simulink subsystem "Batter_Pack_Sim"  (R2022b)
settings: Solver=VariableStepAuto  StartTime=0.0  StopTime=10.0  RelTol=1e-3
undefined symbols (not defined in the file or in its folder): BATT, C, Ion, Lithium, R
libraries: spsIdealSwitchLib x9, spsParallelRLCBranchLib x6, spsBatteryLib x3
settings Model: Creator=MAAM  LastModifiedBy=MAAM

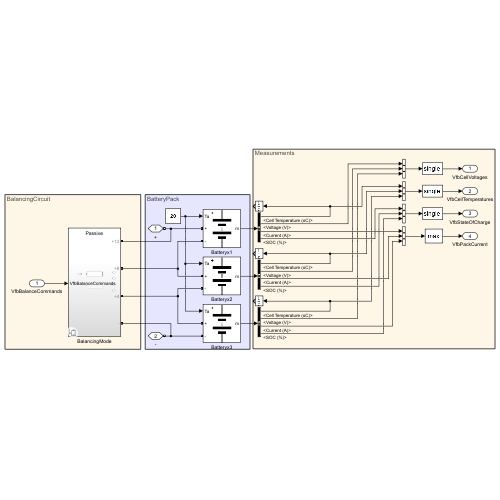
[thumbnail: Simulink's stored preview of the top-level diagram]
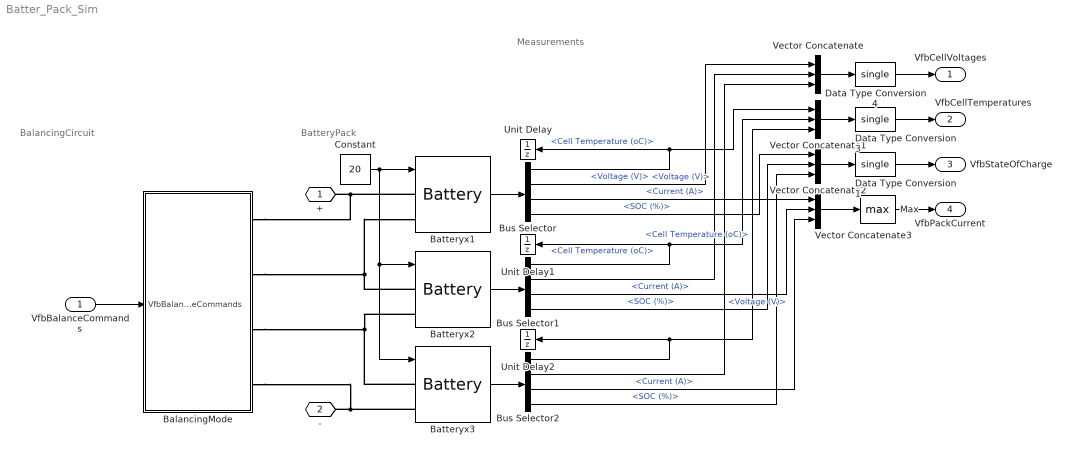
== system Batter_Pack_Sim ==
  note: BalancingCircuit
  note: Measurements
  note: BatteryPack
  VfbBalanceCommands : Inport
  BalancingMode : Subsystem  Variant=on
  Batteryx1 : spsBatteryLib/Battery  BatType=Lithium-Ion  ShowTempParam=on  ThermalPreset=no  ShowAgeParam=off  NomV=double(BATT.Voltage.NominalVolt)  NomQ=double(BATT.Capacity.Type)  SOC=75  Batt_Tr=30  PresetModel=off  MaxQ=double(BATT.Capacity.Max)  MinV=2.55  FullV=double(BATT.Voltage.Full_Dchrg)  Dis_rate=1.3043  R=double(BATT.Res.R0)  Normal_OP=double(BATT.Capacity.Rate)  expZone="[4     0.34]"  current=[6.5 13 32.5]  Units=Time  Tci=20  NomT=20  T2=-30  MaxQ2=double(BATT.Capacity.Rate)  FullV2=double(BATT.Voltage.Init_Dchrg)  Normal_OP2=2.75  expZone2=[3.25 0.5]  Rca=0.06  ti=1000  Dp=0  Neq0=0  Tsim=1e6  Ta1=25  Qeol=5.4*0.9  Reol=0.013333*1.2  Char_age=[2.3478, 3]  Dis_age=[2.3478, 10]  N1=1500  N2=10500  N3=1000  N4=1400  Ta2=45  N5=950
  Batteryx2 : spsBatteryLib/Battery  BatType=Lithium-Ion  ShowTempParam=on  ThermalPreset=no  ShowAgeParam=off  NomV=double(BATT.Voltage.NominalVolt)  NomQ=double(BATT.Capacity.Type)  SOC=85  Batt_Tr=30  PresetModel=off  MaxQ=double(BATT.Capacity.Max)  MinV=2.55  FullV=double(BATT.Voltage.Full_Dchrg)  Dis_rate=1.3043  R=double(BATT.Res.R0)  Normal_OP=double(BATT.Capacity.Rate)  expZone="[4     0.34]"  current=[6.5 13 32.5]  Units=Time  Tci=20  NomT=20  T2=-30  MaxQ2=double(BATT.Capacity.Rate)  FullV2=double(BATT.Voltage.Init_Dchrg)  Normal_OP2=2.75  expZone2=[3.25 0.5]  Rca=0.06  ti=1000  Dp=0  Neq0=0  Tsim=1e6  Ta1=25  Qeol=5.4*0.9  Reol=0.013333*1.2  Char_age=[2.3478, 3]  Dis_age=[2.3478, 10]  N1=1500  N2=10500  N3=1000  N4=1400  Ta2=45  N5=950
  Batteryx3 : spsBatteryLib/Battery  BatType=Lithium-Ion  ShowTempParam=on  ThermalPreset=no  ShowAgeParam=off  NomV=double(BATT.Voltage.NominalVolt)  NomQ=double(BATT.Capacity.Type)  SOC=65  Batt_Tr=30  PresetModel=off  MaxQ=double(BATT.Capacity.Max)  MinV=2.55  FullV=double(BATT.Voltage.Full_Dchrg)  Dis_rate=1.3043  R=double(BATT.Res.R0)  Normal_OP=double(BATT.Capacity.Rate)  expZone="[4     0.34]"  current=[6.5 13 32.5]  Units=Time  Tci=20  NomT=20  T2=-30  MaxQ2=double(BATT.Capacity.Rate)  FullV2=double(BATT.Voltage.Init_Dchrg)  Normal_OP2=2.75  expZone2=[3.25 0.5]  Rca=0.06  ti=1000  Dp=0  Neq0=0  Tsim=1e6  Ta1=25  Qeol=5.4*0.9  Reol=0.013333*1.2  Char_age=[2.3478, 3]  Dis_age=[2.3478, 10]  N1=1500  N2=10500  N3=1000  N4=1400  Ta2=45  N5=950
  Bus Selector : BusSelector  OutputSignals=Cell Temperature (oC),Voltage (V),Current (A),SOC (%)
  Bus Selector1 : BusSelector  OutputSignals=Cell Temperature (oC),Voltage (V),Current (A),SOC (%)
  Bus Selector2 : BusSelector  OutputSignals=Cell Temperature (oC),Voltage (V),Current (A),SOC (%)
  Constant : Constant  Value=20
  Data Type Conversion1 : DataTypeConversion  OutDataTypeStr=single  SaturateOnIntegerOverflow=off  RndMeth=Floor
  Data Type Conversion3 : DataTypeConversion  OutDataTypeStr=single  SaturateOnIntegerOverflow=off  RndMeth=Floor
  Data Type Conversion4 : DataTypeConversion  OutDataTypeStr=single  SaturateOnIntegerOverflow=off  RndMeth=Floor
  Max : MinMax  Function=max  OutDataTypeStr=single
  Unit Delay : UnitDelay  InitialCondition=20  SampleTime=-1  HasFrameUpgradeWarning=on
  Unit Delay1 : UnitDelay  InitialCondition=20  SampleTime=-1  HasFrameUpgradeWarning=on
  Unit Delay2 : UnitDelay  InitialCondition=20  SampleTime=-1  HasFrameUpgradeWarning=on
  Vector Concatenate{,1..3} (4 alike) : Concatenate  NumInputs=3
  + : PMIOPort  Side=Left
  - : PMIOPort  Port=2  Side=Left
  VfbCellVoltages : Outport
  VfbCellTemperatures : Outport  Port=2
  VfbStateOfCharge : Outport  Port=3
  VfbPackCurrent : Outport  Port=4
  wires:
  Constant/1 -> Batteryx2/1, Batteryx3/1, Batteryx1/1
  Data Type Conversion4/1 -> VfbCellVoltages/1
  Data Type Conversion3/1 -> VfbCellTemperatures/1
  Data Type Conversion1/1 -> VfbStateOfCharge/1
  Max/1 -> VfbPackCurrent/1
  Bus Selector1/3 -> Vector Concatenate3/2  "<Current (A)>"
  Bus Selector2/1 -> Vector Concatenate1/3, Unit Delay2/1  "<Cell Temperature (oC)>"
  Bus Selector1/2 -> Vector Concatenate/2  "<Voltage (V)>"
  Vector Concatenate3/1 -> Max/1
  Batteryx1/1 -> Bus Selector/1
  Bus Selector1/4 -> Vector Concatenate2/2  "<SOC (%)>"
  Bus Selector1/1 -> Vector Concatenate1/2, Unit Delay1/1  "<Cell Temperature (oC)>"
  Batteryx3/1 -> Bus Selector2/1
  Bus Selector/4 -> Vector Concatenate2/1  "<SOC (%)>"
  Vector Concatenate2/1 -> Data Type Conversion1/1
  Vector Concatenate/1 -> Data Type Conversion4/1
  Bus Selector2/4 -> Vector Concatenate2/3  "<SOC (%)>"
  Bus Selector/2 -> Vector Concatenate/1  "<Voltage (V)>"
  Bus Selector/3 -> Vector Concatenate3/1  "<Current (A)>"
  Vector Concatenate1/1 -> Data Type Conversion3/1
  Bus Selector2/3 -> Vector Concatenate3/3  "<Current (A)>"
  Batteryx2/1 -> Bus Selector1/1
  Bus Selector2/2 -> Vector Concatenate/3  "<Voltage (V)>"
  Bus Selector/1 -> Vector Concatenate1/1, Unit Delay/1  "<Cell Temperature (oC)>"
  VfbBalanceCommands/1 -> BalancingMode/1(VfbBalanceCommands)
  connections:
  +/RConn1 -- Batteryx1/LConn1 -- BalancingMode/RConn1
  Batteryx3/LConn1 -- BalancingMode/RConn3 -- Batteryx2/LConn2
  Batteryx2/LConn1 -- BalancingMode/RConn2 -- Batteryx1/LConn2
  Batteryx3/LConn2 -- BalancingMode/RConn4 -- -/RConn1

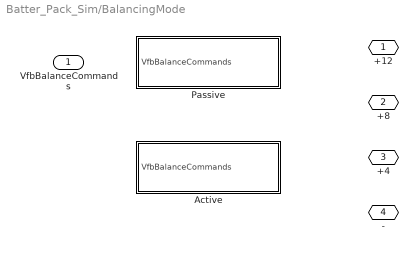
== system Batter_Pack_Sim/BalancingMode ==
  VfbBalanceCommands : Inport
  Active : Subsystem  VariantControl=BATT.Balancing.Mode == BMS_BalMode_Enum.BMS_Active
  Passive : Subsystem  VariantControl=BATT.Balancing.Mode == BMS_BalMode_Enum.BMS_Passive
  +12 : PMIOPort  Side=Right
  +8 : PMIOPort  Port=2  Side=Right
  +4 : PMIOPort  Port=3  Side=Right
  - : PMIOPort  Port=4  Side=Right

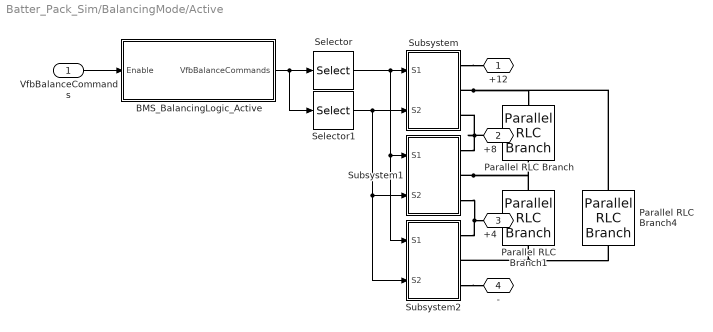
== system Batter_Pack_Sim/BalancingMode/Active ==
  VfbBalanceCommands : Inport
  BMS_BalancingLogic_Active : Stateflow chart  TreatAsAtomicUnit=on
  Parallel RLC Branch : spsParallelRLCBranchLib/Parallel RLC Branch  LConnTagsString=a  RConnTagsString=__new0  BranchType=C  Resistance=1  Inductance=1e-3  SetiL0=off  InitialCurrent=0  Capacitance=C  Setx0=off  InitialVoltage=0  Measurements=None
  Parallel RLC Branch1 : spsParallelRLCBranchLib/Parallel RLC Branch  LConnTagsString=a  RConnTagsString=__new0  BranchType=C  Resistance=1  Inductance=1e-3  SetiL0=off  InitialCurrent=0  Capacitance=C  Setx0=off  InitialVoltage=0  Measurements=None
  Parallel RLC Branch4 : spsParallelRLCBranchLib/Parallel RLC Branch  LConnTagsString=a  RConnTagsString=__new0  BranchType=C  Resistance=1  Inductance=1e-3  SetiL0=off  InitialCurrent=0  Capacitance=C  Setx0=off  InitialVoltage=0  Measurements=None
  Selector : Selector  InputPortWidth=3  IndexOptions=Index vector (dialog)  Indices=1  OutputSizes=1
  Selector1 : Selector  InputPortWidth=3  IndexOptions=Index vector (dialog)  Indices=2  OutputSizes=1
  Subsystem : Subsystem
  Subsystem1 : Subsystem
  Subsystem2 : Subsystem
  +12 : PMIOPort  Side=Right
  +8 : PMIOPort  Port=2  Side=Right
  +4 : PMIOPort  Port=3  Side=Right
  - : PMIOPort  Port=4  Side=Right
  wires:
  Selector1/1 -> Subsystem/2(S2), Subsystem1/2(S2), Subsystem2/2(S2)
  BMS_BalancingLogic_Active/1(VfbBalanceCommands) -> Selector1/1, Selector/1
  Selector/1 -> Subsystem2/1(S1), Subsystem1/1(S1), Subsystem/1(S1)
  VfbBalanceCommands/1 -> BMS_BalancingLogic_Active/1(Enable)
  connections:
  Subsystem1/RConn2 -- Parallel RLC Branch1/LConn1 -- Parallel RLC Branch/RConn1
  Subsystem1/RConn3 -- Subsystem2/RConn1 -- +4/RConn1
  Subsystem/RConn2 -- Parallel RLC Branch4/LConn1 -- Parallel RLC Branch/LConn1
  +8/RConn1 -- Subsystem/RConn3 -- Subsystem1/RConn1
  Parallel RLC Branch1/RConn1 -- Parallel RLC Branch4/RConn1 -- Subsystem2/RConn2
  Subsystem2/RConn3 -- -/RConn1
  Subsystem/RConn1 -- +12/RConn1

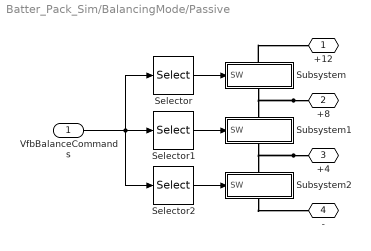
== system Batter_Pack_Sim/BalancingMode/Passive ==
  VfbBalanceCommands : Inport
  Selector : Selector  InputPortWidth=3  IndexOptions=Index vector (dialog)  Indices=1  OutputSizes=1
  Selector1 : Selector  InputPortWidth=3  IndexOptions=Index vector (dialog)  Indices=2  OutputSizes=1
  Selector2 : Selector  InputPortWidth=3  IndexOptions=Index vector (dialog)  Indices=3  OutputSizes=1
  Subsystem : Subsystem
      settings: PortSchema="{\"entries\":[{\"content\":{\"sides\":[{\"content\":{\"connectorIds\":[\"LConn1\"]},\"type\":\"ConnectorPlacement.EquallySpacedRectSide\",\"uuid\":\"eb8fffcd-a71c-4890-8fe1-844de9bb7049\"},{\"content\":{\"connectorIds\":[\"RConn1\"],\"side\":\"RIGHT\"},\"type\":\"ConnectorPlacement.EquallySpacedRectSide\",\"uuid\":\"5d4b0459-fb12-4785-8c10-98c9b0dba58c\"},{\"content\":{\"connectorIds\":[],\"side\":\"TOP\"},\"type\":\"ConnectorPlacement.EquallySpacedRectSide\",\"uuid\":\"54a7a206-2e51-43a0-a96b-a7248b1ad494\"},{\"content\":{\"connectorIds\":[\"In1\"],\"side\":\"BOTTOM\"},\"type\":\"ConnectorPlacement.EquallySpacedRectSide\",\"uuid\":\"fc2549f3-9c78-4be1-a150-7df7a886db86\"}]},\"type\":\"ConnectorPlacement.EquallySpacedConnector\",\"uuid\":\"ba80d02d-3106-485f-afc0-f5d68efbd5a7\"}],\"packageUris\":[\"http://schema.mathworks.com/mf0/Connector/R2020b\"],\"version\":\"1.0\"}"
  Subsystem1 : Subsystem
      settings: PortSchema="{\"entries\":[{\"content\":{\"sides\":[{\"content\":{\"connectorIds\":[\"LConn1\"]},\"type\":\"ConnectorPlacement.EquallySpacedRectSide\",\"uuid\":\"eb8fffcd-a71c-4890-8fe1-844de9bb7049\"},{\"content\":{\"connectorIds\":[\"RConn1\"],\"side\":\"RIGHT\"},\"type\":\"ConnectorPlacement.EquallySpacedRectSide\",\"uuid\":\"5d4b0459-fb12-4785-8c10-98c9b0dba58c\"},{\"content\":{\"connectorIds\":[],\"side\":\"TOP\"},\"type\":\"ConnectorPlacement.EquallySpacedRectSide\",\"uuid\":\"54a7a206-2e51-43a0-a96b-a7248b1ad494\"},{\"content\":{\"connectorIds\":[\"In1\"],\"side\":\"BOTTOM\"},\"type\":\"ConnectorPlacement.EquallySpacedRectSide\",\"uuid\":\"e038b7f9-73dc-4924-8410-20e90d9da844\"}]},\"type\":\"ConnectorPlacement.EquallySpacedConnector\",\"uuid\":\"ba80d02d-3106-485f-afc0-f5d68efbd5a7\"}],\"packageUris\":[\"http://schema.mathworks.com/mf0/Connector/R2020b\"],\"version\":\"1.0\"}"
  Subsystem2 : Subsystem
      settings: PortSchema="{\"entries\":[{\"content\":{\"sides\":[{\"content\":{\"connectorIds\":[\"LConn1\"]},\"type\":\"ConnectorPlacement.EquallySpacedRectSide\",\"uuid\":\"eb8fffcd-a71c-4890-8fe1-844de9bb7049\"},{\"content\":{\"connectorIds\":[\"RConn1\"],\"side\":\"RIGHT\"},\"type\":\"ConnectorPlacement.EquallySpacedRectSide\",\"uuid\":\"5d4b0459-fb12-4785-8c10-98c9b0dba58c\"},{\"content\":{\"connectorIds\":[],\"side\":\"TOP\"},\"type\":\"ConnectorPlacement.EquallySpacedRectSide\",\"uuid\":\"54a7a206-2e51-43a0-a96b-a7248b1ad494\"},{\"content\":{\"connectorIds\":[\"In1\"],\"side\":\"BOTTOM\"},\"type\":\"ConnectorPlacement.EquallySpacedRectSide\",\"uuid\":\"f8f2bbaf-62e5-4d8f-96ff-782bcab3079c\"}]},\"type\":\"ConnectorPlacement.EquallySpacedConnector\",\"uuid\":\"ba80d02d-3106-485f-afc0-f5d68efbd5a7\"}],\"packageUris\":[\"http://schema.mathworks.com/mf0/Connector/R2020b\"],\"version\":\"1.0\"}"
  +12 : PMIOPort  Side=Right
  +8 : PMIOPort  Port=2  Side=Right
  +4 : PMIOPort  Port=3  Side=Right
  - : PMIOPort  Port=4  Side=Right
  wires:
  VfbBalanceCommands/1 -> Selector2/1, Selector/1, Selector1/1
  Selector/1 -> Subsystem/1(SW)
  Selector1/1 -> Subsystem1/1(SW)
  Selector2/1 -> Subsystem2/1(SW)
  connections:
  +4/RConn1 -- Subsystem2/LConn1 -- Subsystem1/RConn1
  +8/RConn1 -- Subsystem1/LConn1 -- Subsystem/RConn1
  Subsystem/LConn1 -- +12/RConn1
  Subsystem2/RConn1 -- -/RConn1

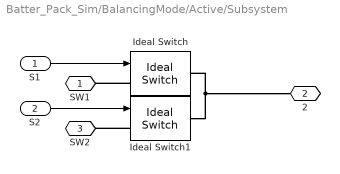
== system Batter_Pack_Sim/BalancingMode/Active/Subsystem ==
  S1 : Inport
  S2 : Inport  Port=2
  Ideal Switch : spsIdealSwitchLib/Ideal Switch  Ron=0.0001  Lon=0  IC=0  Rs=1e7  Cs=inf  Measurements=off
  Ideal Switch1 : spsIdealSwitchLib/Ideal Switch  Ron=0.0001  Lon=0  IC=0  Rs=1e7  Cs=inf  Measurements=off
  SW1 : PMIOPort  Side=Right
  2 : PMIOPort  Port=2  Side=Right
  SW2 : PMIOPort  Port=3  Side=Right
  wires:
  S1/1 -> Ideal Switch/1
  S2/1 -> Ideal Switch1/1
  connections:
  Ideal Switch1/RConn1 -- 2/RConn1 -- Ideal Switch/RConn1
  Ideal Switch/LConn1 -- SW1/RConn1
  Ideal Switch1/LConn1 -- SW2/RConn1

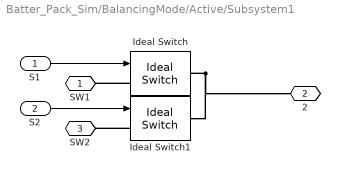
== system Batter_Pack_Sim/BalancingMode/Active/Subsystem1 ==
  S1 : Inport
  S2 : Inport  Port=2
  Ideal Switch : spsIdealSwitchLib/Ideal Switch  Ron=0.0001  Lon=0  IC=0  Rs=1e7  Cs=inf  Measurements=off
  Ideal Switch1 : spsIdealSwitchLib/Ideal Switch  Ron=0.0001  Lon=0  IC=0  Rs=1e7  Cs=inf  Measurements=off
  SW1 : PMIOPort  Side=Right
  2 : PMIOPort  Port=2  Side=Right
  SW2 : PMIOPort  Port=3  Side=Right
  wires:
  S2/1 -> Ideal Switch1/1
  S1/1 -> Ideal Switch/1
  connections:
  Ideal Switch1/LConn1 -- SW2/RConn1
  Ideal Switch/LConn1 -- SW1/RConn1
  Ideal Switch/RConn1 -- 2/RConn1 -- Ideal Switch1/RConn1

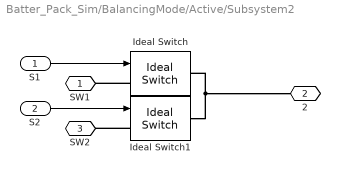
== system Batter_Pack_Sim/BalancingMode/Active/Subsystem2 ==
  S1 : Inport
  S2 : Inport  Port=2
  Ideal Switch : spsIdealSwitchLib/Ideal Switch  Ron=0.0001  Lon=0  IC=0  Rs=1e7  Cs=inf  Measurements=off
  Ideal Switch1 : spsIdealSwitchLib/Ideal Switch  Ron=0.0001  Lon=0  IC=0  Rs=1e7  Cs=inf  Measurements=off
  SW1 : PMIOPort  Side=Right
  2 : PMIOPort  Port=2  Side=Right
  SW2 : PMIOPort  Port=3  Side=Right
  wires:
  S1/1 -> Ideal Switch/1
  S2/1 -> Ideal Switch1/1
  connections:
  Ideal Switch1/RConn1 -- 2/RConn1 -- Ideal Switch/RConn1
  Ideal Switch/LConn1 -- SW1/RConn1
  Ideal Switch1/LConn1 -- SW2/RConn1

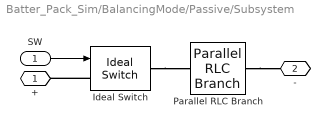
== system Batter_Pack_Sim/BalancingMode/Passive/Subsystem ==
  SW : Inport
  Ideal Switch : spsIdealSwitchLib/Ideal Switch  Ron=0.001  Lon=0  IC=0  Rs=1e5  Cs=inf  Measurements=off
  Parallel RLC Branch : spsParallelRLCBranchLib/Parallel RLC Branch  LConnTagsString=a  RConnTagsString=__new0  BranchType=R  Resistance=R  Inductance=1e-3  SetiL0=off  InitialCurrent=0  Capacitance=1e-6  Setx0=off  InitialVoltage=0  Measurements=None
  + : PMIOPort  Side=Left
  - : PMIOPort  Port=2  Side=Right
  wires:
  SW/1 -> Ideal Switch/1
  connections:
  Ideal Switch/LConn1 -- +/RConn1
  Ideal Switch/RConn1 -- Parallel RLC Branch/LConn1
  Parallel RLC Branch/RConn1 -- -/RConn1

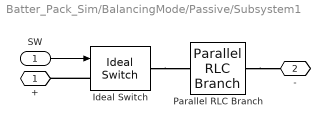
== system Batter_Pack_Sim/BalancingMode/Passive/Subsystem1 ==
  SW : Inport
  Ideal Switch : spsIdealSwitchLib/Ideal Switch  Ron=0.001  Lon=0  IC=0  Rs=1e5  Cs=inf  Measurements=off
  Parallel RLC Branch : spsParallelRLCBranchLib/Parallel RLC Branch  LConnTagsString=a  RConnTagsString=__new0  BranchType=R  Resistance=R  Inductance=1e-3  SetiL0=off  InitialCurrent=0  Capacitance=1e-6  Setx0=off  InitialVoltage=0  Measurements=None
  + : PMIOPort  Side=Left
  - : PMIOPort  Port=2  Side=Right
  wires:
  SW/1 -> Ideal Switch/1
  connections:
  Parallel RLC Branch/RConn1 -- -/RConn1
  Ideal Switch/RConn1 -- Parallel RLC Branch/LConn1
  Ideal Switch/LConn1 -- +/RConn1

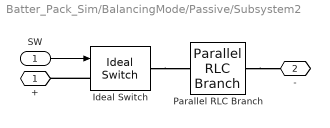
== system Batter_Pack_Sim/BalancingMode/Passive/Subsystem2 ==
  SW : Inport
  Ideal Switch : spsIdealSwitchLib/Ideal Switch  Ron=0.001  Lon=0  IC=0  Rs=1e5  Cs=inf  Measurements=off
  Parallel RLC Branch : spsParallelRLCBranchLib/Parallel RLC Branch  LConnTagsString=a  RConnTagsString=__new0  BranchType=R  Resistance=R  Inductance=1e-3  SetiL0=off  InitialCurrent=0  Capacitance=1e-6  Setx0=off  InitialVoltage=0  Measurements=None
  + : PMIOPort  Side=Left
  - : PMIOPort  Port=2  Side=Right
  wires:
  SW/1 -> Ideal Switch/1
  connections:
  Ideal Switch/LConn1 -- +/RConn1
  Ideal Switch/RConn1 -- Parallel RLC Branch/LConn1
  Parallel RLC Branch/RConn1 -- -/RConn1

== stateflow chart Batter_Pack_Sim/BalancingMode/Active/BMS_BalancingLogic_Active ==
  state WaitEnable
    en:
    VfbBalanceCommands(:,:) = false;
  state BalancingActiveMode
    state SW1_On
      en:
      VfbBalanceCommands(1) = true;
      ex:
      VfbBalanceCommands(1) = false;
      step = 1;
    state SW_Wait
    state SW2_On
      en:
      VfbBalanceCommands(2) = true;
      ex:
      VfbBalanceCommands(2) = false;
      step = 2;
    (default) -> SW1_On
    SW_Wait -> SW1_On [order 1] : after((0.5-Don)/Freq, sec)[step >= 2]
    SW1_On -> SW_Wait : after(Don/Freq - 0.0001, sec)
    SW_Wait -> SW2_On [order 2] : after((0.5-Don)/Freq, sec)[step <= 1]
    SW2_On -> SW_Wait : after(Don/Freq - 0.0001, sec)
  (default) -> WaitEnable
  WaitEnable -> BalancingActiveMode : [any(Enable)]
  BalancingActiveMode -> WaitEnable : [~any(Enable)]
  data: VfbBalanceCommands output boolean size=BATT.Package.Ns_Module*BATT.Package.NumModules =boolean(zeros(1,BATT.Package.Ns_Module*BATT.Package.NumModules))'; Don constant single size=1 =BATT.Balancing.Duty; Freq constant single size=1 =BATT.Balancing.Freq; BalancingThreshold_ON constant single size=1 =BATT.Balancing.ThresholdOn; step local single size=1 =single(1); BalancingOffWait constant uint8 size=1 =BATT.Balancing.BalWaitOff; BalancingOnWait constant uint8 size=1 =BATT.Balancing.BalWaitOn; BalancingFlag local boolean size=1 =true; BalancingMode constant boolean size=1 =BATT.Balancing.Mode; BalancingThreshold_OFF constant single size=1 =BATT.Balancing.ThresholdOff; Enable input
